simulink model "lab6"  (Simulink 10.0)
settings: Solver=ode4  StartTime=0.0  StopTime=0.4  RelTol=1e-3
settings Model: Creator=16ara3  LastModifiedBy=ameanasad
settings DataIOCC: SaveFormat=Dataset  ReturnWorkspaceOutputs=on
settings OptimizationCC: LifeSpan=auto
settings DebuggingCC: UnderspecifiedInitializationDetection=Simplified  MergeDetectMultiDrivingBlocksExec=error  SFUnexpectedBacktrackingDiag=error  SFNoUnconditionalDefaultTransitionDiag=error  SFExecutionAtInitializationDiag=warning  ArithmeticOperatorsInVariantConditions=error
settings HardwareCC: ProdBitPerPointer=64  ProdBitPerSizeT=64  ProdBitPerPtrDiffT=64  ProdLargestAtomicFloat=Float  ProdIntDivRoundTo=Zero  ProdEndianess=LittleEndian  ProdWordSize=64  ProdHWDeviceType=Intel->x86-64 (Windows64)
settings ModelReferenceCC: PropagateSignalLabelsOutOfModel=on
settings SFSimCC: SimUseLocalCustomCode=on
settings RTWCC: RTWUseLocalCustomCode=on
settings CodeAppCC: StateflowObjectComments=off
settings GRTTargetCC: TargetLangStandard=C99 (ISO)  CombineOutputUpdateFcns=on  GRTInterface=off
settings ConfigComp: CovMetricSettings=dwe  CovHtmlReporting=off  CovSaveCumulativeToWorkspaceVar=off  CovSaveSingleToWorkspaceVar=off

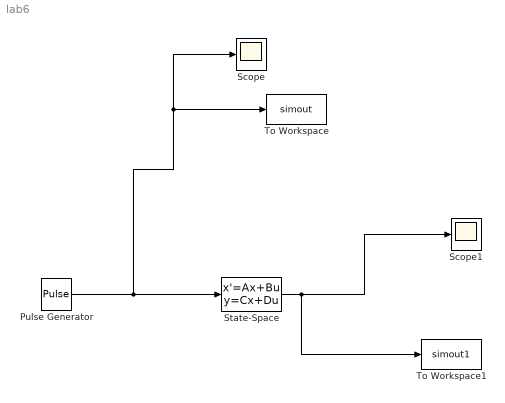
== system lab6 ==
  Pulse Generator : DiscretePulseGenerator  PulseType=Time based  Amplitude=5  Period=10.0  PulseWidth=(0.2/10)*10  VectorParams1D=off
  Scope : Scope
  Scope1 : Scope
  State-Space : StateSpace  A=[0, 1; 0, -1/0.034]  B=[0; 220.58]  C=[0, 1]  D=[0]  InitialCondition=[0, 0]
  To Workspace : ToWorkspace  VariableName=simout  SaveFormat=Structure With Time  SampleTime=-1
  To Workspace1 : ToWorkspace  VariableName=simout1  SaveFormat=Structure With Time  SampleTime=-1
  wires:
  Pulse Generator/1 -> Scope/1, To Workspace/1, State-Space/1
  State-Space/1 -> To Workspace1/1, Scope1/1
